simulink model "Control_System_Testbench_V2"  (R2018b)
settings: Solver=VariableStepAuto  StartTime=0.0  StopTime=100  RelTol=1e-3  EnableMultiTasking=on
undefined symbols (not defined in the file): Jw, R, sigbuilder_block
settings Model: Creator=univ4123  LastModifiedBy=univ4123
settings OptimizationCC: LifeSpan=inf
settings DebuggingCC: SFUnexpectedBacktrackingDiag=warning  SFNoUnconditionalDefaultTransitionDiag=warning
settings SFSimCC: SimUseLocalCustomCode=off
settings RTWCC: RTWUseLocalCustomCode=off
settings CodeAppCC: StateflowObjectComments=on
settings GRTTargetCC: TargetLangStandard=C89/C90 (ANSI)  GeneratePreprocessorConditionals=Disable all
settings ConfigComp: CovMetricSettings=dw  CovHtmlReporting=on  CovSaveCumulativeToWorkspaceVar=on  CovSaveSingleToWorkspaceVar=on  CovExternalEMLEnable=off

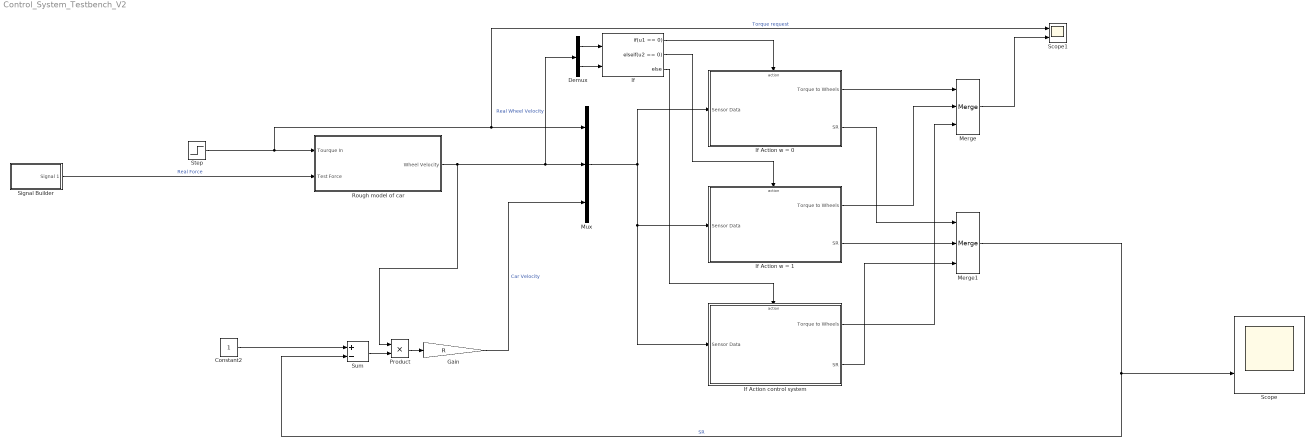
== system Control_System_Testbench_V2 ==
  Constant2 : Constant  SampleTime=0.1
  Demux : Demux  Outputs=2
  Gain : Gain  Gain=R
  If : If  NumInputs=2  IfExpression=u1 == 0  ElseIfExpressions=u2 == 0
  If Action control system : Subsystem  TreatAsAtomicUnit=on
  If Action w = 0 : Subsystem  TreatAsAtomicUnit=on
  If Action w = 1 : Subsystem  TreatAsAtomicUnit=on
  Merge : Merge  Inputs=3
  Merge1 : Merge  Inputs=3
  Mux : Mux  Inputs=3
  Product : Product
  Rough model of car : Subsystem
  Scope : Scope  NumInputPorts=2
  Scope1 : Scope  NumInputPorts=2
  Signal Builder : Subsystem  Tag=STV Subsys  LoadFcn=sigbuilder_block('load');  StartFcn=sigbuilder_block('start');  StopFcn=sigbuilder_block('stop');  ClipboardFcn=sigbuilder_block('clipboard');  mask(Sigbuilder block){tuvar=[0:10]}
      mask help: Simulink:masks:SigbuilderBlock_MD
      mask init:
      | if ~strcmp(get_param(bdroot(gcbh),'SimulationStatus'),'stopped') tuvar = sigbuilder_block('maskInit'); end
      settings: CopyFcn=sigbuilder_block('copy');  DeleteFcn=sigbuilder_block('delete');  ModelCloseFcn=sigbuilder_block('modelClose');  PreSaveFcn=sigbuilder_block('preSave');  PauseFcn=sigbuilder_block('pause');  ContinueFcn=sigbuilder_block('continue');  NameChangeFcn=sigbuilder_block('namechange');  OpenFcn=sigbuilder_block('open',[437.6 153.75 550.4 359.25 ]);  CloseFcn=sigbuilder_block('close');
      mask Display: plot(0, 0, 100, 100,[2, 2, 32, 32, 2], [68, 8, 8, 68, 68],[32, 2], [38, 38], [32, 19, 2],[53, 60, 44], [32, 17, 17, 2],[16, 16, 31, 31]);txt = getActiveGroup(gcbh);text(2, 100, txt,'verticalAlignment', 'top');
  Step : Step  After=5  SampleTime=0.1
  Sum : Sum  Inputs=+-
  wires:
  Step/1 -> Scope1/1, Mux/1, Rough model of car/1(Tourque In)  "Torque request"
  Rough model of car/1(Wheel Velocity) -> Demux/1, Mux/2, Product/1  "Real Wheel Velocity"
  Gain/1 -> Mux/3  "Car Velocity"
  Merge1/1 -> Sum/2, Scope/2  "SR"
  Signal Builder/1(Signal 1) -> Rough model of car/2(Test Force)  "Real Force"
  Constant2/1 -> Sum/1
  Sum/1 -> Product/2
  Product/1 -> Gain/1
  Merge/1 -> Scope1/2
  Mux/1 -> If Action control system/1(Sensor Data), If Action w = 1/1(Sensor Data), If Action w = 0/1(Sensor Data)
  If Action w = 0/1(Torque to Wheels) -> Merge/1
  If Action control system/1(Torque to Wheels) -> Merge/3
  If Action w = 0/2(SR) -> Merge1/1
  If Action control system/2(SR) -> Merge1/3
  Demux/1 -> If/1
  Demux/2 -> If/2
  If Action w = 1/1(Torque to Wheels) -> Merge/2
  If Action w = 1/2(SR) -> Merge1/2
  If/1 -> If Action w = 0/Action
  If/2 -> If Action w = 1/Action
  If/3 -> If Action control system/Action

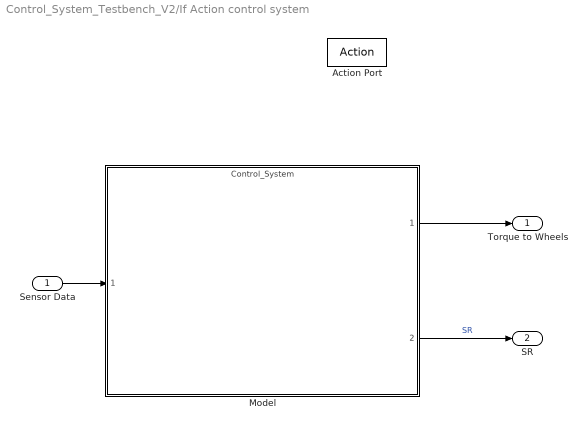
== system Control_System_Testbench_V2/If Action control system ==
  Sensor Data : Inport
  Action Port : ActionPort  ActionType=else
  Model : ModelReference  ModelNameDialog=Control_System.slx  SimulationMode=Normal  ModelReferenceVersion=1.17
  Torque to Wheels : Outport
  SR : Outport  Port=2
  wires:
  Sensor Data/1 -> Model/1
  Model/1 -> Torque to Wheels/1
  Model/2 -> SR/1  "SR"

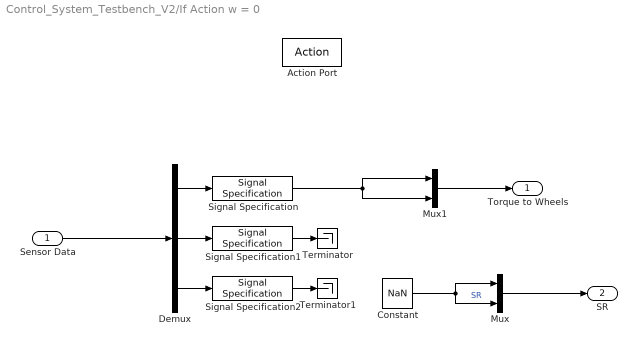
== system Control_System_Testbench_V2/If Action w = 0 ==
  Sensor Data : Inport
  Action Port : ActionPort  ActionType=then
  Constant : Constant  Value=NaN
  Demux : Demux  Outputs=3
  Mux : Mux  Inputs=2
  Mux1 : Mux  Inputs=2
  Signal Specification : SignalSpecification  Dimensions=1
  Signal Specification1 : SignalSpecification  Dimensions=2
  Signal Specification2 : SignalSpecification  Dimensions=2
  Terminator : Terminator
  Terminator1 : Terminator
  Torque to Wheels : Outport
  SR : Outport  Port=2
  wires:
  Constant/1 -> Mux/2, Mux/1  "SR"
  Sensor Data/1 -> Demux/1
  Demux/1 -> Signal Specification/1
  Demux/2 -> Signal Specification1/1
  Demux/3 -> Signal Specification2/1
  Mux/1 -> SR/1
  Signal Specification2/1 -> Terminator1/1
  Signal Specification1/1 -> Terminator/1
  Signal Specification/1 -> Mux1/2, Mux1/1
  Mux1/1 -> Torque to Wheels/1

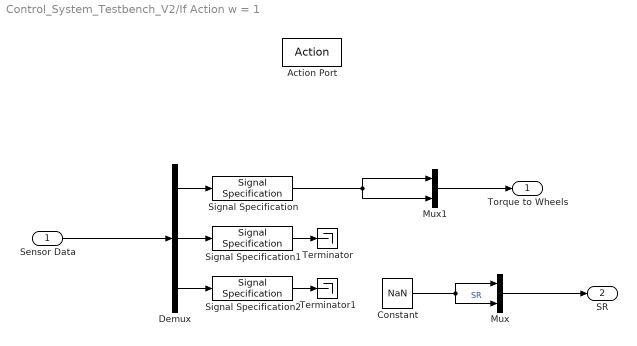
== system Control_System_Testbench_V2/If Action w = 1 ==
  Sensor Data : Inport
  Action Port : ActionPort  ActionType=elseif
  Constant : Constant  Value=NaN
  Demux : Demux  Outputs=3
  Mux : Mux  Inputs=2
  Mux1 : Mux  Inputs=2
  Signal Specification : SignalSpecification  Dimensions=1
  Signal Specification1 : SignalSpecification  Dimensions=2
  Signal Specification2 : SignalSpecification  Dimensions=2
  Terminator : Terminator
  Terminator1 : Terminator
  Torque to Wheels : Outport
  SR : Outport  Port=2
  wires:
  Constant/1 -> Mux/2, Mux/1  "SR"
  Sensor Data/1 -> Demux/1
  Demux/1 -> Signal Specification/1
  Demux/2 -> Signal Specification1/1
  Demux/3 -> Signal Specification2/1
  Mux/1 -> SR/1
  Signal Specification2/1 -> Terminator1/1
  Signal Specification1/1 -> Terminator/1
  Signal Specification/1 -> Mux1/2, Mux1/1
  Mux1/1 -> Torque to Wheels/1

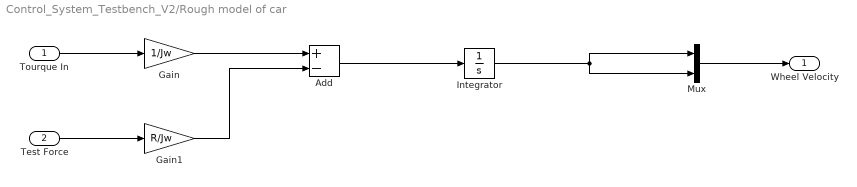
== system Control_System_Testbench_V2/Rough model of car ==
  Tourque In : Inport
  Test Force : Inport  Port=2
  Add : Sum  Inputs=+-
  Gain : Gain  Gain=1/Jw
  Gain1 : Gain  Gain=R/Jw
  Integrator : Integrator
  Mux : Mux  Inputs=2
  Wheel Velocity : Outport
  wires:
  Tourque In/1 -> Gain/1
  Gain/1 -> Add/1
  Test Force/1 -> Gain1/1
  Add/1 -> Integrator/1
  Gain1/1 -> Add/2
  Mux/1 -> Wheel Velocity/1
  Integrator/1 -> Mux/1, Mux/2

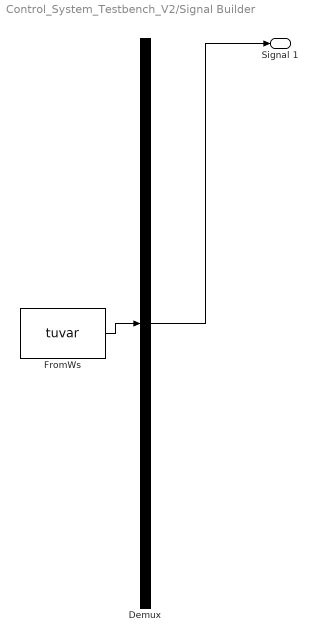
== system Control_System_Testbench_V2/Signal Builder ==
  Demux : Demux  Tag=STV Demux  Outputs=1
  FromWs : FromWorkspace  Tag=STV FromWs  VariableName=tuvar  SampleTime=0
      SigBuilderData=|
      | common.afterFinalStr = 'Extrapolate'
      | common.sampleTime = 0
      | dataSet.timeRange = [0 10]
      | dataSet.name = 'Group 1'
      | sbobj.Groups.Name = 'Group 1'
      | sbobj.Groups.Signals.Name = 'Signal 1'
      | sbobj.Groups.Signals.XData = [0 1 4 6 7 10]
      | sbobj.Groups.Signals.YData = [0 0 9.9 4.3 2.05 0]
  Signal 1 : Outport  Tag=STV Outport
  wires:
  Demux/1 -> Signal 1/1
  FromWs/1 -> Demux/1
